simulink model "kalman_w_error"  (R2013b)
settings: Solver=FixedStepDiscrete  StartTime=10  StopTime=200  FixedStep=0.05  RelTol=1e-3
settings Model: Creator=Franta  LastModifiedBy=Franta

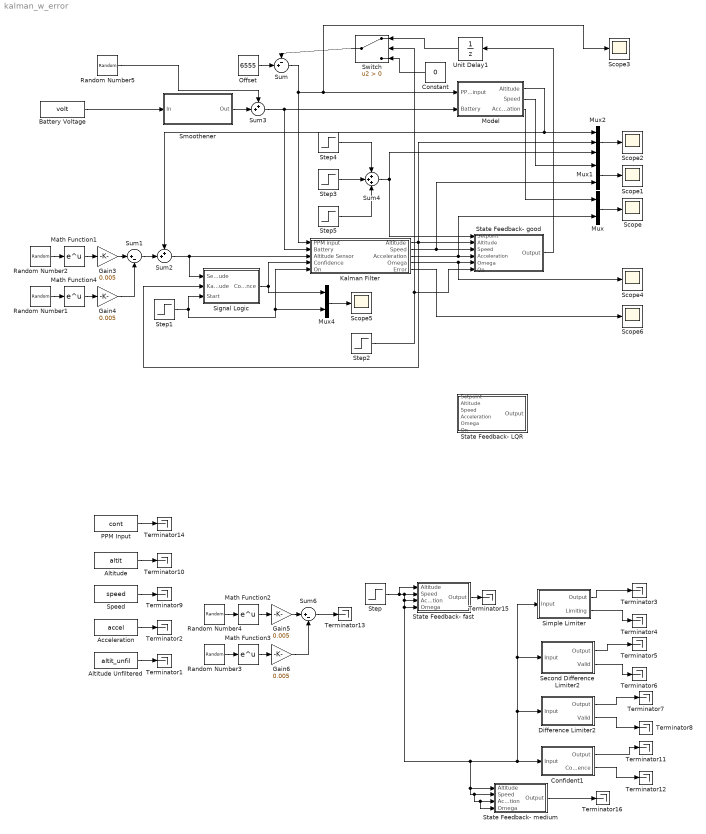
== system kalman_w_error ==
  Acceleration : FromWorkspace  VariableName=accel  SampleTime=0  OutputAfterFinalValue=Holding final value
  Altitude : FromWorkspace  VariableName=altit  SampleTime=0  OutputAfterFinalValue=Holding final value
  Altitude Unfiltered : FromWorkspace  VariableName=altit_unfil  SampleTime=0  OutputAfterFinalValue=Holding final value
  Battery Voltage : FromWorkspace  VariableName=volt  SampleTime=0  OutputAfterFinalValue=Holding final value
  Confident1 : Subsystem
  Constant : Constant  Value=0
  Difference Limiter2 : Subsystem
  Gain{3..6} (4 alike) : Gain  Gain=0.005
  Kalman Filter : Subsystem
  Math Function{1..4} (4 alike) : Math  SaturateOnIntegerOverflow=on
  Model : Subsystem
  Mux : Mux  Inputs=2
  Mux1 : Mux  Inputs=2
  Mux2 : Mux  Inputs=3
  Mux4 : Mux  Inputs=2
  Offset : Constant  Value=6555
  PPM Input : FromWorkspace  VariableName=cont  SampleTime=0  OutputAfterFinalValue=Holding final value
  Random Number1 : RandomNumber  Variance=4  Seed=1  SampleTime=0.05
  Random Number2 : RandomNumber  Variance=4  SampleTime=0.05
  Random Number3 : RandomNumber  Variance=4  Seed=1  SampleTime=0.05
  Random Number4 : RandomNumber  Variance=4  SampleTime=0.05
  Random Number5 : RandomNumber  Variance=0.01  Seed=3  SampleTime=0.05
  Scope{,1..6} (7 alike) : Scope
      Scope settings: YMin=0  YMax=47.5
      Scope1 settings: TimeRange=50
      Scope2 settings: SaveName=ScopeData2
      Scope3 settings: SaveName=ScopeData3
      Scope4 settings: YMin=0  YMax=47.5  SaveName=ScopeData4
      Scope5 settings: SaveName=ScopeData5
      Scope6 settings: YMin=0  YMax=47.5  SaveName=ScopeData6
  Second Difference Limiter2 : Subsystem
  Signal Logic : Subsystem
  Simple Limiter : Subsystem
  Smoothener : Subsystem
  Speed : FromWorkspace  VariableName=speed  SampleTime=0  OutputAfterFinalValue=Holding final value
  State Feedback- LQR : Subsystem
  State Feedback- fast : Subsystem
  State Feedback- good : Subsystem
  State Feedback- medium : Subsystem
  Step : Step  Time=150  SampleTime=0
  Step1 : Step  Time=10.1  SampleTime=0
  Step2 : Step  Time=21.5  SampleTime=0
  Step3 : Step  Time=100  SampleTime=0
  Step4 : Step  Time=21.5  SampleTime=0
  Step5 : Step  Time=150  After=-1  SampleTime=0
  Sum : Sum  Inputs=-+|
  Sum1 : Sum  Inputs=|+-
  Sum2 : Sum  Inputs=++|
  Sum3 : Sum  Inputs=++|
  Sum4 : Sum  Inputs=+++
  Sum6 : Sum  Inputs=|+-
  Switch : Switch  Criteria=u2 > Threshold
  Terminator{1..16} (16 alike) : Terminator
  Unit Delay1 : UnitDelay  SampleTime=-1
  wires:
  Mux/1 -> Scope/1
  Mux1/1 -> Scope1/1
  Mux2/1 -> Scope2/1
  Kalman Filter/3(Acceleration) -> State Feedback- good/4(Acceleration), Mux/2
  Simple Limiter/1(Output) -> Terminator3/1
  Simple Limiter/2(Limiting) -> Terminator4/1
  Second Difference Limiter2/1(Output) -> Terminator5/1
  Second Difference Limiter2/2(Valid) -> Terminator6/1
  Difference Limiter2/1(Output) -> Terminator7/1
  Difference Limiter2/2(Valid) -> Terminator8/1
  Kalman Filter/2(Speed) -> State Feedback- good/3(Speed), Mux1/2
  Confident1/1(Output) -> Terminator11/1
  Confident1/2(Confidence) -> Terminator12/1
  Sum2/1 -> Signal Logic/1(Sensor Altitude), Kalman Filter/3(Altitude Sensor)
  Sum4/1 -> State Feedback- good/1(Setpoint), Mux2/3
  Step/1 -> State Feedback- fast/3(Acceleration), State Feedback- fast/4(Omega), State Feedback- medium/4(Omega), State Feedback- medium/3(Acceleration), State Feedback- medium/2(Speed), State Feedback- medium/1(Altitude), Simple Limiter/1(Input), Second Difference Limiter2/1(Input), Difference Limiter2/1(Input), Confident1/1(Input), State Feedback- fast/2(Speed), State Feedback- fast/1(Altitude)
  State Feedback- medium/1(Output) -> Terminator16/1
  State Feedback- fast/1(Output) -> Terminator15/1
  Kalman Filter/4(Omega) -> State Feedback- good/5(Omega), Scope4/1
  Model/1(Altitude) -> Sum2/1, Mux2/1
  Model/2(Speed) -> Mux1/1
  Model/3(Acceleration) -> Mux/1
  Altitude Unfiltered/1 -> Terminator1/1
  Sum1/1 -> Sum2/2
  Random Number4/1 -> Math Function2/1
  Math Function2/1 -> Gain5/1
  Random Number3/1 -> Math Function3/1
  Math Function3/1 -> Gain6/1
  Gain6/1 -> Sum6/2
  Gain5/1 -> Sum6/1
  Sum6/1 -> Terminator13/1
  Acceleration/1 -> Terminator2/1
  Speed/1 -> Terminator9/1
  Altitude/1 -> Terminator10/1
  Random Number2/1 -> Math Function1/1
  Math Function1/1 -> Gain3/1
  Random Number1/1 -> Math Function4/1
  Math Function4/1 -> Gain4/1
  Gain4/1 -> Sum1/2
  Gain3/1 -> Sum1/1
  State Feedback- good/1(Output) -> Unit Delay1/1
  Offset/1 -> Sum/2
  Sum/1 -> Kalman Filter/1(PPM input), Scope3/1, Model/1(PPM input)
  Mux4/1 -> Scope5/1
  Kalman Filter/1(Altitude) -> State Feedback- good/2(Altitude), Mux2/2, Signal Logic/2(Kalman Altitude)
  Signal Logic/1(Confidence) -> Mux4/1, Kalman Filter/4(Confidence)
  Step1/1 -> Kalman Filter/5(On), Mux4/2, Signal Logic/3(Start)
  PPM Input/1 -> Terminator14/1
  Kalman Filter/5(Error) -> Scope6/1
  Switch/1 -> Sum/1
  Unit Delay1/1 -> Switch/1
  Constant/1 -> Switch/3
  Step2/1 -> State Feedback- good/6(On), Switch/2
  Battery Voltage/1 -> Smoothener/1(In)
  Smoothener/1(Out) -> Sum3/2
  Sum3/1 -> Kalman Filter/2(Battery), Model/2(Battery)
  Random Number5/1 -> Sum3/1
  Step3/1 -> Sum4/2
  Step4/1 -> Sum4/1
  Step5/1 -> Sum4/3

== system kalman_w_error/Confident1 ==
  Input : Inport
  MATLAB Function : MATLAB Function  TreatAsAtomicUnit=on
  Threshold : Constant  Value=0.35
  Unit Delay : UnitDelay  InitialCondition=0.5  SampleTime=-1
  Unit Delay1 : UnitDelay  SampleTime=-1
  Output : Outport
  Confidence : Outport  Port=2
  wires:
  Unit Delay1/1 -> MATLAB Function/4(cycles)
  MATLAB Function/3(cyclesBlind) -> Unit Delay1/1
  MATLAB Function/2(confidence) -> Confidence/1
  Unit Delay/1 -> MATLAB Function/3(lastGood)
  MATLAB Function/1(good) -> Unit Delay/1
  Threshold/1 -> MATLAB Function/2(threshold)
  Input/1 -> MATLAB Function/1(input), Output/1

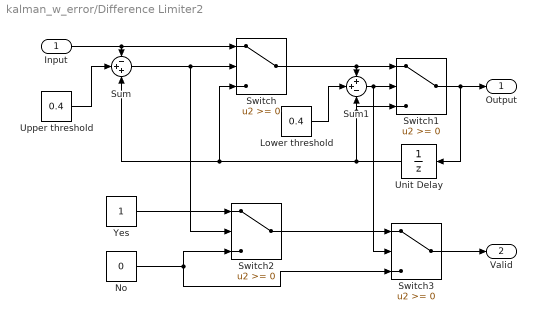
== system kalman_w_error/Difference Limiter2 ==
  Input : Inport
  Lower threshold : Constant  Value=0.4
  No : Constant  Value=0
  Sum : Sum  Inputs=-++
  Sum1 : Sum  Inputs=++-
  Switch{,1..3} (4 alike) : Switch
  Unit Delay : UnitDelay  InitialCondition=1  SampleTime=-1
  Upper threshold : Constant  Value=0.4
  Yes : Constant
  Output : Outport
  Valid : Outport  Port=2
  wires:
  Lower threshold/1 -> Sum1/2
  Switch/1 -> Switch1/1, Sum1/1
  Switch1/1 -> Unit Delay/1, Output/1
  Upper threshold/1 -> Sum/2
  Input/1 -> Switch/1, Sum/1
  Unit Delay/1 -> Sum/3, Switch/3, Switch1/3, Sum1/3
  Sum/1 -> Switch2/2, Switch/2
  Sum1/1 -> Switch3/2, Switch1/2
  Yes/1 -> Switch2/1
  No/1 -> Switch2/3, Switch3/3
  Switch2/1 -> Switch3/1
  Switch3/1 -> Valid/1

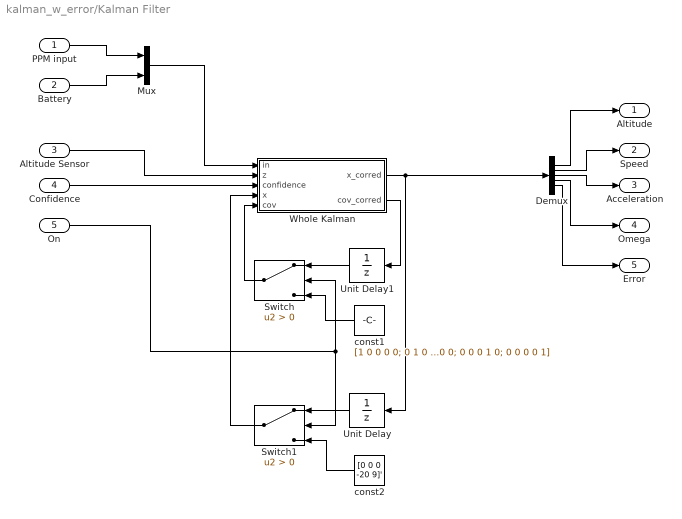
== system kalman_w_error/Kalman Filter ==
  PPM input : Inport
  Battery : Inport  Port=2
  Altitude Sensor : Inport  Port=3
  Confidence : Inport  Port=4
  On : Inport  Port=5
  Demux : Demux  Outputs=5
  Mux : Mux  Inputs=2
  Switch : Switch  Criteria=u2 > Threshold
  Switch1 : Switch  Criteria=u2 > Threshold
  Unit Delay : UnitDelay  InitialCondition=[0 0 0 0 0]'  SampleTime=-1
  Unit Delay1 : UnitDelay  InitialCondition=[1 0 0 0 0; 0 1 0 0 0; 0 0 1 0 0; 0 0 0 1 0; 0 0 0 0 1]  SampleTime=-1
  Whole Kalman : MATLAB Function  TreatAsAtomicUnit=on
  const1 : Constant  Value=[1 0 0 0 0; 0 1 0 0 0; 0 0 1 0 0; 0 0 0 1 0; 0 0 0 0 1]
  const2 : Constant  Value=[0 0 0 -20 9]'
  Altitude : Outport
  Speed : Outport  Port=2
  Acceleration : Outport  Port=3
  Omega : Outport  Port=4
  Error : Outport  Port=5
  wires:
  Whole Kalman/1(x_corred) -> Demux/1, Unit Delay/1
  Mux/1 -> Whole Kalman/1(in)
  PPM input/1 -> Mux/1
  Battery/1 -> Mux/2
  Demux/2 -> Speed/1
  Demux/3 -> Acceleration/1
  Demux/1 -> Altitude/1
  Demux/4 -> Omega/1
  Whole Kalman/2(cov_corred) -> Unit Delay1/1
  Confidence/1 -> Whole Kalman/3(confidence)
  Altitude Sensor/1 -> Whole Kalman/2(z)
  Unit Delay1/1 -> Switch/1
  Switch/1 -> Whole Kalman/5(cov)
  Unit Delay/1 -> Switch1/1
  Switch1/1 -> Whole Kalman/4(x)
  const1/1 -> Switch/3
  const2/1 -> Switch1/3
  On/1 -> Switch/2, Switch1/2
  Demux/5 -> Error/1

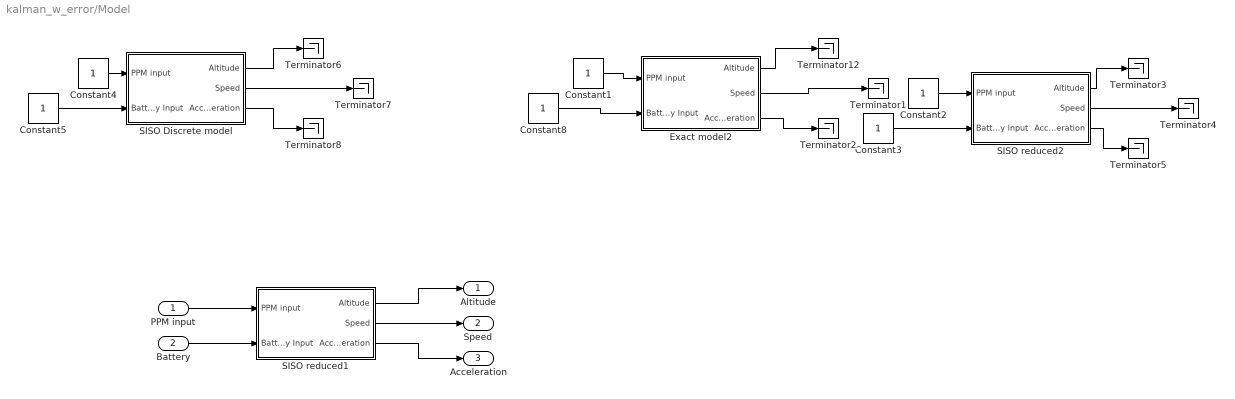
== system kalman_w_error/Model ==
  PPM input : Inport
  Battery : Inport  Port=2
  Constant{1..5,8} (6 alike) : Constant
  Exact model2 : Subsystem
  SISO Discrete model : Subsystem
  SISO reduced1 : Subsystem
  SISO reduced2 : Subsystem
  Terminator{1..8,12} (9 alike) : Terminator
  Altitude : Outport
  Speed : Outport  Port=2
  Acceleration : Outport  Port=3
  wires:
  SISO reduced2/1(Altitude) -> Terminator3/1
  SISO reduced2/2(Speed) -> Terminator4/1
  SISO reduced2/3(Acceleration) -> Terminator5/1
  Constant3/1 -> SISO reduced2/2(Battery Input)
  Constant2/1 -> SISO reduced2/1(PPM input)
  SISO Discrete model/1(Altitude) -> Terminator6/1
  SISO Discrete model/2(Speed) -> Terminator7/1
  SISO Discrete model/3(Acceleration) -> Terminator8/1
  Constant5/1 -> SISO Discrete model/2(Battery Input)
  Constant4/1 -> SISO Discrete model/1(PPM input)
  Constant8/1 -> Exact model2/2(Battery Input)
  Constant1/1 -> Exact model2/1(PPM input)
  Exact model2/1(Altitude) -> Terminator12/1
  Exact model2/2(Speed) -> Terminator1/1
  Exact model2/3(Acceleration) -> Terminator2/1
  PPM input/1 -> SISO reduced1/1(PPM input)
  Battery/1 -> SISO reduced1/2(Battery Input)
  SISO reduced1/1(Altitude) -> Altitude/1
  SISO reduced1/2(Speed) -> Speed/1
  SISO reduced1/3(Acceleration) -> Acceleration/1

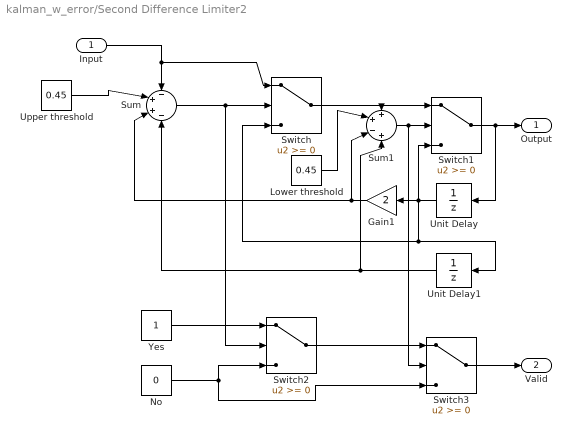
== system kalman_w_error/Second Difference Limiter2 ==
  Input : Inport
  Gain1 : Gain  Gain=2
  Lower threshold : Constant  Value=0.45
  No : Constant  Value=0
  Sum : Sum  Inputs=-++-
  Sum1 : Sum  Inputs=++-+
  Switch{,1..3} (4 alike) : Switch
  Unit Delay : UnitDelay  InitialCondition=1  SampleTime=-1
  Unit Delay1 : UnitDelay  InitialCondition=1  SampleTime=-1
  Upper threshold : Constant  Value=0.45
  Yes : Constant
  Output : Outport
  Valid : Outport  Port=2
  wires:
  Gain1/1 -> Sum1/3, Sum/3
  Switch3/1 -> Valid/1
  Switch2/1 -> Switch3/1
  No/1 -> Switch3/3, Switch2/3
  Yes/1 -> Switch2/1
  Sum1/1 -> Switch1/2, Switch3/2
  Sum/1 -> Switch2/2, Switch/2
  Unit Delay/1 -> Gain1/1, Switch1/3, Unit Delay1/1, Switch/3
  Input/1 -> Switch/1, Sum/1
  Upper threshold/1 -> Sum/2
  Switch1/1 -> Output/1, Unit Delay/1
  Switch/1 -> Switch1/1, Sum1/1
  Lower threshold/1 -> Sum1/2
  Unit Delay1/1 -> Sum1/4, Sum/4

== system kalman_w_error/Signal Logic ==
  Sensor Altitude : Inport
  Kalman Altitude : Inport  Port=2
  Start : Inport  Port=3
  Confident : Subsystem
  Required Fit : Constant  Value=0.4
  Required Fit1 : Constant
  Starter : Subsystem
  Switch : Switch  Criteria=u2 > Threshold
  Confidence : Outport
  wires:
  Sensor Altitude/1 -> Starter/1(Sensor Altitude), Confident/1(Input)
  Start/1 -> Starter/3(Start)
  Switch/1 -> Confidence/1
  Required Fit/1 -> Starter/4(Required Fit)
  Kalman Altitude/1 -> Starter/2(Kalman Altitude)
  Starter/1(Confidence Override) -> Switch/2
  Confident/1(Confidence) -> Switch/3
  Required Fit1/1 -> Switch/1

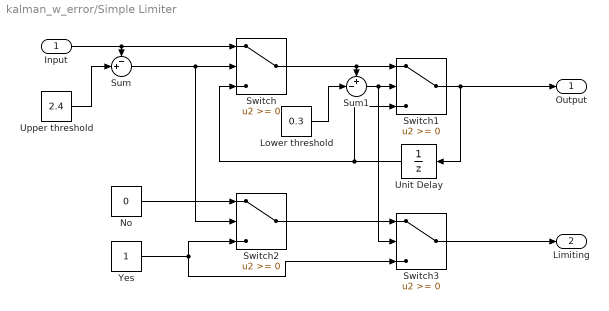
== system kalman_w_error/Simple Limiter ==
  Input : Inport
  Lower threshold : Constant  Value=0.3
  No : Constant  Value=0
  Sum : Sum  Inputs=-+|
  Sum1 : Sum  Inputs=+-|
  Switch{,1..3} (4 alike) : Switch
  Unit Delay : UnitDelay  SampleTime=-1
  Upper threshold : Constant  Value=2.4
  Yes : Constant
  Output : Outport
  Limiting : Outport  Port=2
  wires:
  Unit Delay/1 -> Switch1/3, Switch/3
  Sum/1 -> Switch2/2, Switch/2
  Input/1 -> Sum/1, Switch/1
  Upper threshold/1 -> Sum/2
  Switch1/1 -> Output/1, Unit Delay/1
  Sum1/1 -> Switch3/2, Switch1/2
  Switch/1 -> Sum1/1, Switch1/1
  Lower threshold/1 -> Sum1/2
  No/1 -> Switch2/1
  Yes/1 -> Switch2/3, Switch3/3
  Switch2/1 -> Switch3/1
  Switch3/1 -> Limiting/1

== system kalman_w_error/Smoothener ==
  In : Inport
  Demux : Demux  Outputs=20
  Gain : Gain  Gain=0.05
  Mux : Mux  Inputs=20
  Sum of Elements : Sum  Inputs=+
  Terminator : Terminator
  Unit Delay : UnitDelay  InitialCondition=[11.7 11.7 11.7 11.7 11.7 11.7 11.7 11.7 11.7 11.7 11.7 11.7 11.7 11.7 11.7 11.7 11.7 11.7 11.7 11.7]  SampleTime=-1
  Out : Outport
  wires:
  In/1 -> Mux/1
  Demux/1 -> Mux/2
  Demux/2 -> Mux/3
  Demux/3 -> Mux/4
  Demux/4 -> Mux/5
  Mux/1 -> Unit Delay/1, Sum of Elements/1
  Sum of Elements/1 -> Gain/1
  Gain/1 -> Out/1
  Unit Delay/1 -> Demux/1
  Demux/5 -> Mux/6
  Demux/6 -> Mux/7
  Demux/7 -> Mux/8
  Demux/8 -> Mux/9
  Demux/9 -> Mux/10
  Demux/10 -> Mux/11
  Demux/11 -> Mux/12
  Demux/12 -> Mux/13
  Demux/13 -> Mux/14
  Demux/14 -> Mux/15
  Demux/15 -> Mux/16
  Demux/16 -> Mux/17
  Demux/17 -> Mux/18
  Demux/18 -> Mux/19
  Demux/19 -> Mux/20
  Demux/20 -> Terminator/1

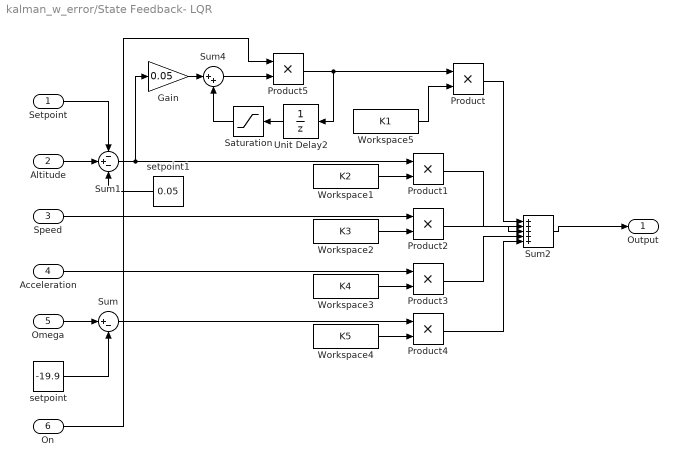
== system kalman_w_error/State Feedback- LQR ==
  Setpoint : Inport
  Altitude : Inport  Port=2
  Speed : Inport  Port=3
  Acceleration : Inport  Port=4
  Omega : Inport  Port=5
  On : Inport  Port=6
  Gain : Gain  Gain=0.05
  Product{,1..5} (6 alike) : Product
  Saturation : Saturate  UpperLimit=100  LowerLimit=-100
  Sum : Sum  Inputs=|+-
  Sum1 : Sum  Inputs=-+-
  Sum2 : Sum  Inputs=+++++
  Sum4 : Sum  Inputs=|++
  Unit Delay2 : UnitDelay  SampleTime=-1
  Workspace1 : FromWorkspace  VariableName=K2  Interpolate=off  OutputAfterFinalValue=Holding final value
  Workspace2 : FromWorkspace  VariableName=K3  Interpolate=off  OutputAfterFinalValue=Holding final value
  Workspace3 : FromWorkspace  VariableName=K4  Interpolate=off  OutputAfterFinalValue=Holding final value
  Workspace4 : FromWorkspace  VariableName=K5  Interpolate=off  OutputAfterFinalValue=Holding final value
  Workspace5 : FromWorkspace  VariableName=K1  Interpolate=off  OutputAfterFinalValue=Holding final value
  setpoint : Constant  Value=-19.9
  setpoint1 : Constant  Value=0.05
  Output : Outport
  wires:
  setpoint1/1 -> Sum1/3
  On/1 -> Product5/1
  Product5/1 -> Unit Delay2/1, Product/1
  Sum4/1 -> Product5/2
  Product4/1 -> Sum2/5
  Workspace5/1 -> Product/2
  Sum2/1 -> Output/1
  Omega/1 -> Sum/1
  Altitude/1 -> Sum1/2
  Sum1/1 -> Gain/1, Product1/1
  Setpoint/1 -> Sum1/1
  Saturation/1 -> Sum4/2
  Unit Delay2/1 -> Saturation/1
  Workspace1/1 -> Product1/2
  Workspace2/1 -> Product2/2
  Workspace4/1 -> Product4/2
  Sum/1 -> Product4/1
  Product2/1 -> Sum2/3
  Product1/1 -> Sum2/2
  Product3/1 -> Sum2/4
  Product/1 -> Sum2/1
  setpoint/1 -> Sum/2
  Acceleration/1 -> Product3/1
  Speed/1 -> Product2/1
  Workspace3/1 -> Product3/2
  Gain/1 -> Sum4/1

== system kalman_w_error/State Feedback- fast ==
  Altitude : Inport
  Speed : Inport  Port=2
  Acceleration : Inport  Port=3
  Omega : Inport  Port=4
  Gain : Gain  Gain=652.0
  Gain1 : Gain  Gain=1322.8
  Gain2 : Gain  Gain=-238.1
  Gain3 : Gain  Gain=1238.2
  Sum : Sum  Inputs=++++
  Output : Outport
  wires:
  Altitude/1 -> Gain/1
  Speed/1 -> Gain1/1
  Acceleration/1 -> Gain2/1
  Omega/1 -> Gain3/1
  Gain/1 -> Sum/1
  Gain1/1 -> Sum/2
  Gain2/1 -> Sum/3
  Gain3/1 -> Sum/4
  Sum/1 -> Output/1

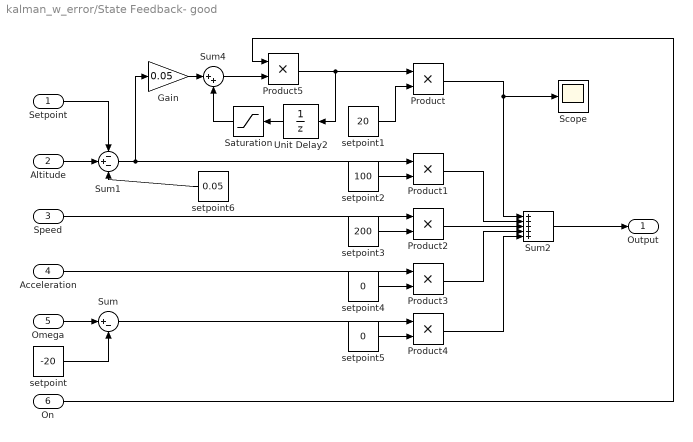
== system kalman_w_error/State Feedback- good ==
  Setpoint : Inport
  Altitude : Inport  Port=2
  Speed : Inport  Port=3
  Acceleration : Inport  Port=4
  Omega : Inport  Port=5
  On : Inport  Port=6
  Gain : Gain  Gain=0.05
  Product{,1..5} (6 alike) : Product
  Saturation : Saturate  UpperLimit=100  LowerLimit=-100
  Scope : Scope
      settings: SaveName=ScopeData7
  Sum : Sum  Inputs=|+-
  Sum1 : Sum  Inputs=-+-
  Sum2 : Sum  Inputs=+++++
  Sum4 : Sum  Inputs=|++
  Unit Delay2 : UnitDelay  SampleTime=-1
  setpoint : Constant  Value=-20
  setpoint1 : Constant  Value=20
  setpoint2 : Constant  Value=100
  setpoint3 : Constant  Value=200
  setpoint4 : Constant  Value=0
  setpoint5 : Constant  Value=0
  setpoint6 : Constant  Value=0.05
  Output : Outport
  wires:
  Gain/1 -> Sum4/1
  setpoint4/1 -> Product3/2
  Speed/1 -> Product2/1
  Acceleration/1 -> Product3/1
  setpoint/1 -> Sum/2
  Product4/1 -> Sum2/5
  Product/1 -> Sum2/1, Scope/1
  Product3/1 -> Sum2/4
  Product1/1 -> Sum2/2
  Product2/1 -> Sum2/3
  Sum/1 -> Product4/1
  setpoint5/1 -> Product4/2
  setpoint3/1 -> Product2/2
  setpoint2/1 -> Product1/2
  Unit Delay2/1 -> Saturation/1
  Saturation/1 -> Sum4/2
  Setpoint/1 -> Sum1/1
  Sum1/1 -> Product1/1, Gain/1
  Altitude/1 -> Sum1/2
  Omega/1 -> Sum/1
  Sum2/1 -> Output/1
  setpoint1/1 -> Product/2
  Product5/1 -> Unit Delay2/1, Product/1
  Sum4/1 -> Product5/2
  On/1 -> Product5/1
  setpoint6/1 -> Sum1/3

== system kalman_w_error/State Feedback- medium ==
  Altitude : Inport
  Speed : Inport  Port=2
  Acceleration : Inport  Port=3
  Omega : Inport  Port=4
  Gain : Gain  Gain=475.6
  Gain1 : Gain  Gain=972.8
  Gain2 : Gain  Gain=-281.7
  Gain3 : Gain  Gain=1002.8
  Sum : Sum  Inputs=++++
  Output : Outport
  wires:
  Sum/1 -> Output/1
  Gain3/1 -> Sum/4
  Gain2/1 -> Sum/3
  Gain1/1 -> Sum/2
  Gain/1 -> Sum/1
  Omega/1 -> Gain3/1
  Acceleration/1 -> Gain2/1
  Speed/1 -> Gain1/1
  Altitude/1 -> Gain/1

== system kalman_w_error/Model/Exact model2 ==
  PPM input : Inport
  Battery Input : Inport  Port=2
  Demux : Demux
  Discrete State-Space : DiscreteStateSpace  A=[1 0.05 0 0; 0 1 0.05 0; 0 0 0 1; 0 0 -0.65658 1.5714]  B=[0 0 0; 0 0 0; 0.00091141 -0.36830 -2.8005; 0.0011525 -0.052414 -7.5757]  C=[1 0 0 0; 0 1 0 0; 0 0 1 0; 0 0 0 1]  D=[0 0 0; 0 0 0; 0 0 0; 0 0 0]  SampleTime=0.05
  Mux : Mux  Inputs=3
  Terminator : Terminator
  const : Constant
  Altitude : Outport
  Speed : Outport  Port=2
  Acceleration : Outport  Port=3
  wires:
  const/1 -> Mux/3
  Battery Input/1 -> Mux/2
  PPM input/1 -> Mux/1
  Discrete State-Space/1 -> Demux/1
  Demux/3 -> Acceleration/1
  Demux/2 -> Speed/1
  Demux/1 -> Altitude/1
  Mux/1 -> Discrete State-Space/1
  Demux/4 -> Terminator/1

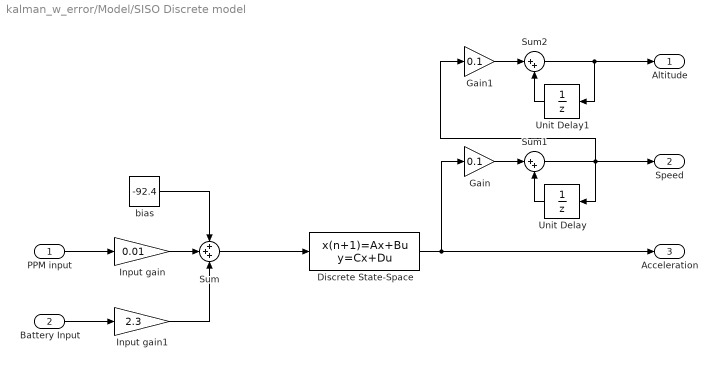
== system kalman_w_error/Model/SISO Discrete model ==
  PPM input : Inport
  Battery Input : Inport  Port=2
  Discrete State-Space : DiscreteStateSpace  A=[0 1; -0.67523 1.64069]  B=[0.28811; 0.18591]  C=[1 0]  D=0  SampleTime=0.1
  Gain : Gain  Gain=0.1
  Gain1 : Gain  Gain=0.1
  Input gain : Gain  Gain=0.01
  Input gain1 : Gain  Gain=2.3
  Sum : Sum  Inputs=+++
  Sum1 : Sum  Inputs=|++
  Sum2 : Sum  Inputs=|++
  Unit Delay : UnitDelay  SampleTime=-1
  Unit Delay1 : UnitDelay  InitialCondition=1  SampleTime=-1
  bias : Constant  Value=-92.4
  Altitude : Outport
  Speed : Outport  Port=2
  Acceleration : Outport  Port=3
  wires:
  PPM input/1 -> Input gain/1
  Battery Input/1 -> Input gain1/1
  Input gain/1 -> Sum/2
  Input gain1/1 -> Sum/3
  bias/1 -> Sum/1
  Sum/1 -> Discrete State-Space/1
  Discrete State-Space/1 -> Gain/1, Acceleration/1
  Unit Delay/1 -> Sum1/2
  Sum1/1 -> Unit Delay/1, Gain1/1, Speed/1
  Sum2/1 -> Unit Delay1/1, Altitude/1
  Unit Delay1/1 -> Sum2/2
  Gain/1 -> Sum1/1
  Gain1/1 -> Sum2/1

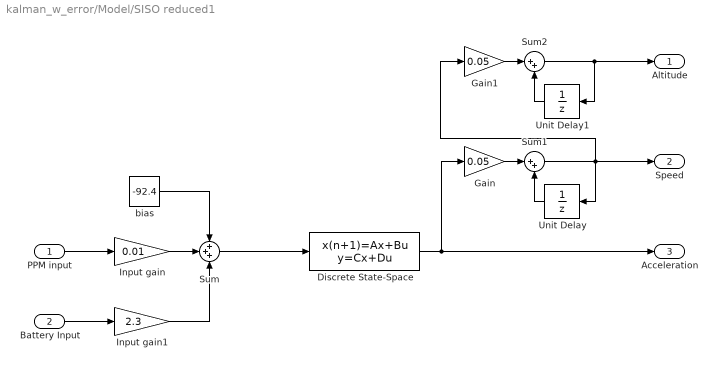
== system kalman_w_error/Model/SISO reduced1 ==
  PPM input : Inport
  Battery Input : Inport  Port=2
  Discrete State-Space : DiscreteStateSpace  A=[0.8379]  B=[0.1382]  C=[1]  D=0  SampleTime=0.05
  Gain : Gain  Gain=0.05
  Gain1 : Gain  Gain=0.05
  Input gain : Gain  Gain=0.01
  Input gain1 : Gain  Gain=2.3
  Sum : Sum  Inputs=+++
  Sum1 : Sum  Inputs=|++
  Sum2 : Sum  Inputs=|++
  Unit Delay : UnitDelay  SampleTime=-1
  Unit Delay1 : UnitDelay  SampleTime=-1
  bias : Constant  Value=-92.4
  Altitude : Outport
  Speed : Outport  Port=2
  Acceleration : Outport  Port=3
  wires:
  PPM input/1 -> Input gain/1
  Battery Input/1 -> Input gain1/1
  Input gain/1 -> Sum/2
  Input gain1/1 -> Sum/3
  bias/1 -> Sum/1
  Sum/1 -> Discrete State-Space/1
  Discrete State-Space/1 -> Gain/1, Acceleration/1
  Unit Delay/1 -> Sum1/2
  Sum1/1 -> Unit Delay/1, Gain1/1, Speed/1
  Sum2/1 -> Unit Delay1/1, Altitude/1
  Unit Delay1/1 -> Sum2/2
  Gain/1 -> Sum1/1
  Gain1/1 -> Sum2/1

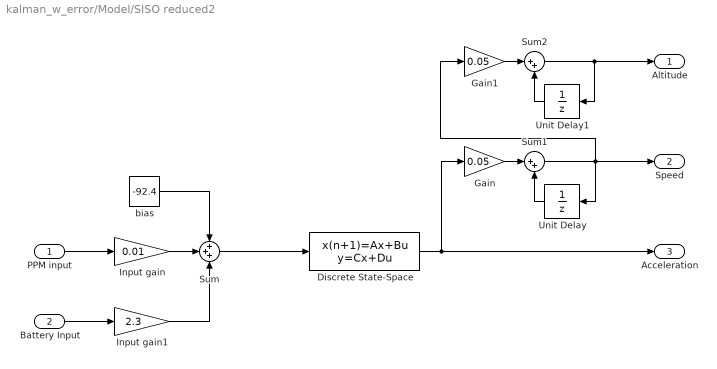
== system kalman_w_error/Model/SISO reduced2 ==
  PPM input : Inport
  Battery Input : Inport  Port=2
  Discrete State-Space : DiscreteStateSpace  A=[0.8379]  B=[0.1382]  C=[1]  D=0  SampleTime=0.05
  Gain : Gain  Gain=0.05
  Gain1 : Gain  Gain=0.05
  Input gain : Gain  Gain=0.01
  Input gain1 : Gain  Gain=2.3
  Sum : Sum  Inputs=+++
  Sum1 : Sum  Inputs=|++
  Sum2 : Sum  Inputs=|++
  Unit Delay : UnitDelay  SampleTime=-1
  Unit Delay1 : UnitDelay  SampleTime=-1
  bias : Constant  Value=-92.4
  Altitude : Outport
  Speed : Outport  Port=2
  Acceleration : Outport  Port=3
  wires:
  Gain1/1 -> Sum2/1
  Gain/1 -> Sum1/1
  Unit Delay1/1 -> Sum2/2
  Sum2/1 -> Altitude/1, Unit Delay1/1
  Sum1/1 -> Speed/1, Gain1/1, Unit Delay/1
  Unit Delay/1 -> Sum1/2
  Discrete State-Space/1 -> Acceleration/1, Gain/1
  Sum/1 -> Discrete State-Space/1
  bias/1 -> Sum/1
  Input gain1/1 -> Sum/3
  Input gain/1 -> Sum/2
  Battery Input/1 -> Input gain1/1
  PPM input/1 -> Input gain/1

== system kalman_w_error/Signal Logic/Confident ==
  Input : Inport
  MATLAB Function : MATLAB Function  TreatAsAtomicUnit=on
  Threshold : Constant  Value=0.35
  Unit Delay : UnitDelay  InitialCondition=0.5  SampleTime=-1
  Unit Delay1 : UnitDelay  SampleTime=-1
  Confidence : Outport
  wires:
  Input/1 -> MATLAB Function/1(input)
  Threshold/1 -> MATLAB Function/2(threshold)
  MATLAB Function/1(good) -> Unit Delay/1
  Unit Delay/1 -> MATLAB Function/3(lastGood)
  MATLAB Function/2(confidence) -> Confidence/1
  MATLAB Function/3(cyclesBlind) -> Unit Delay1/1
  Unit Delay1/1 -> MATLAB Function/4(cycles)

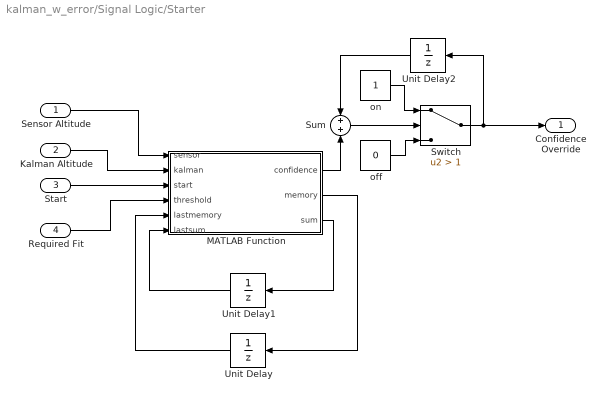
== system kalman_w_error/Signal Logic/Starter ==
  Sensor Altitude : Inport
  Kalman Altitude : Inport  Port=2
  Start : Inport  Port=3
  Required Fit : Inport  Port=4
  MATLAB Function : MATLAB Function  TreatAsAtomicUnit=on
  Sum : Sum  Inputs=+|+
  Switch : Switch  Criteria=u2 > Threshold  Threshold=1
  Unit Delay : UnitDelay  InitialCondition="[0 0 0 0 0 0 0 0 0 0  0 0 0 0 0 0 0 0 0 0]"  SampleTime=-1
  Unit Delay1 : UnitDelay  SampleTime=-1
  Unit Delay2 : UnitDelay  InitialCondition=1  SampleTime=-1
  off : Constant  Value=0
  on : Constant
  Confidence Override : Outport
  wires:
  Sensor Altitude/1 -> MATLAB Function/1(sensor)
  Start/1 -> MATLAB Function/3(start)
  Unit Delay/1 -> MATLAB Function/5(lastmemory)
  Required Fit/1 -> MATLAB Function/4(threshold)
  Kalman Altitude/1 -> MATLAB Function/2(kalman)
  MATLAB Function/2(memory) -> Unit Delay/1
  MATLAB Function/3(sum) -> Unit Delay1/1
  Unit Delay1/1 -> MATLAB Function/6(lastsum)
  MATLAB Function/1(confidence) -> Sum/2
  off/1 -> Switch/3
  on/1 -> Switch/1
  Sum/1 -> Switch/2
  Unit Delay2/1 -> Sum/1
  Switch/1 -> Unit Delay2/1, Confidence Override/1

== matlab function kalman_w_error/Kalman Filter/Whole Kalman ==
  data: in input; z input; confidence input; x_corred output; cov_corred output; x input; cov input
function [x_corred, cov_corred] = kalman(in, z, confidence, x, cov)
u = ((in(1)/100) + (in(2)*2.3));
A = [1 0.05 0 0 0; 0 1 0.05 0 0; 0 0 0 1 1; 0 0 -0.66953 1.58995 0; 0 0 0 0 1];
B = [0; 0; 0.11700; 0.12710; 0];
P = [1 0 0 0 0];
Q = 1000/confidence;
R = [1 0 0 0 0; 0 1 0 0 0; 0 0 1 0 0; 0 0 0 1 0; 0 0 0 0 1];

% prediction
x_next = A*x + B*u;
cov_next = (A*cov*A') + R;

% correction
if (confidence > 0.001)
    K = (cov_next*P')/((P*cov_next*P') + Q);
    x_corred = x_next + K*(z - P*x_next);
    cov_corred = (eye(5) - K*P)*cov_next;
else % do not correct
    x_corred = x_next;
    cov_corred = cov_next;
end

== matlab function kalman_w_error/Confident1/MATLAB Function ==
  data: input input; threshold input; good output; lastGood input; confidence output; cycles input; cyclesBlind output
function [good, confidence, cyclesBlind] = confident(input, threshold, lastGood, cycles)

if (input == lastGood)
    good = lastGood;    
    confidence = 0;
    cyclesBlind = 0;
else
    if (abs(input - lastGood) > threshold)
        if (cycles < 16)
            good = lastGood;
            confidence = (2^cycles)/65536;
            cyclesBlind = cycles + 1;
        else
            good = input;
            confidence = 1;
            cyclesBlind = 0;
        end        
    else
        good = input;
        confidence = 1;
        cyclesBlind = 0;
    end
end

== matlab function kalman_w_error/Signal Logic/Confident/MATLAB Function ==
  data: input input; threshold input; good output; lastGood input; confidence output; cycles input; cyclesBlind output
function [good, confidence, cyclesBlind] = confident(input, threshold, lastGood, cycles)

if (input == lastGood)
        if (cycles < 16)
            good = lastGood;    
            confidence = 1 - (cycles/16)^2;
            cyclesBlind = cycles + 1;
        else
            good = lastGood;  
            confidence = 0;
            cyclesBlind = cycles + 1;
        end     
else
    if (abs(input - lastGood) > threshold)
        if (cycles < 16)
            good = lastGood;
            confidence = (2^cycles)/65536;
            cyclesBlind = cycles + 1;
        else
            good = input;
            confidence = 1;
            cyclesBlind = 0;
        end        
    else
        good = input;
        confidence = 1;
        cyclesBlind = 0;
    end
end

== matlab function kalman_w_error/Signal Logic/Starter/MATLAB Function ==
  data: confidence output; sensor input; kalman input; start input; threshold input; lastmemory input; lastsum input; memory output; sum output
function [confidence, memory, sum] = starter(sensor, kalman, start, threshold, lastmemory, lastsum)

if (start > 0)
    memory = zeros(20, 1);
    memory(1) = abs(sensor - kalman);
    memory(2:20) = lastmemory(1:19);
    sum = lastsum - lastmemory(20) + memory(1);
        if (lastsum > threshold)
            confidence = 1;
        else
            confidence = 0;
        end     
else
    sum = 2;
    memory = 0.1*ones(20, 1);
    confidence = 1;
end
